simulink model "adc16_single_chan"  (R2013a)
settings: Solver=ode45  StartTime=0.0  StopTime=4096  RelTol=1e-3
undefined symbols (not defined in the file): pfb_coeff_gen_calc
libraries: xbsIndex_r4 x2131, casper_library_misc x50, simulink x31, casper_library_delays x18, casper_library_pfbs x4, xps_library x1
(part 1 of 27)
settings Model: Creator=root  LastModifiedBy=root

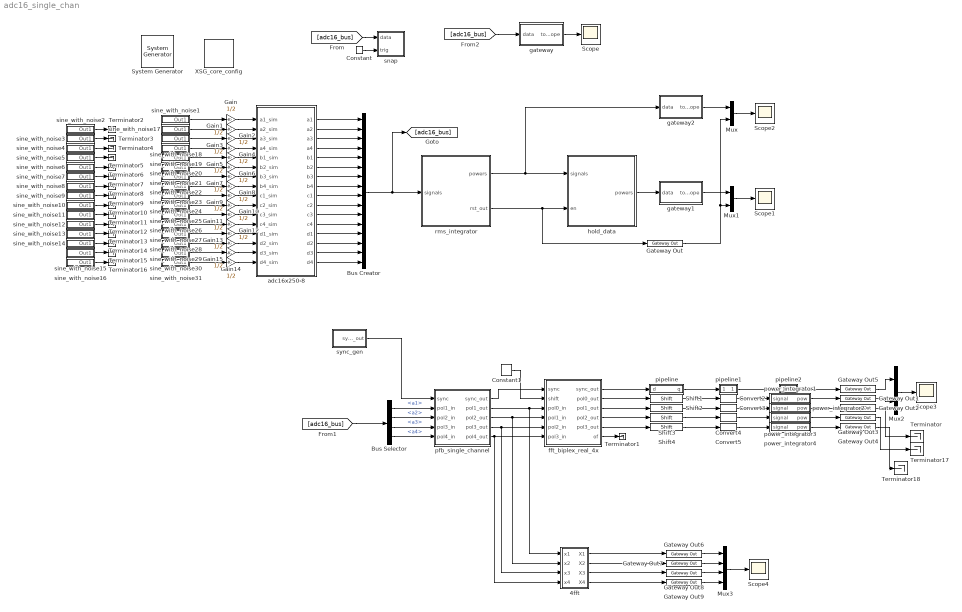
== system adc16_single_chan ==
  " System Generator" : xbsIndex_r4/ System Generator  Tag=genX  xilinxfamily=Kintex7  part=xc7k325t  speed=-3  package=fbg676  synthesis_tool=XST  clock_wrapper=Clock Enables  directory=./netlist  proj_type=Project Navigator  Synth_file=XST Defaults  Impl_file=ISE Defaults  testbench=off  simulink_period=1  sysclk_period=10  dcm_input_clock_period=10  incr_netlist=off  trim_vbits=Everywhere in SubSystem  dbl_ovrd=According to Block Masks  core_generation=According to Block Masks  run_coregen=off  deprecated_control=off  eval_field=0  block_type=sysgen
  4fft : Subsystem
  Bus Creator : BusCreator  Inputs=16
  Bus Selector : BusSelector  OutputSignals=a1,a2,a3,a4
  Constant : xbsIndex_r4/Constant  const=1  gui_display_data_type=Boolean  arith_type=Boolean  n_bits=16  bin_pt=14  preci_type=Single  exp_width=8  frac_width=24  explicit_period=off  period=1  equ=P=C  opselect=C  inp2=PCIN>>17  opr=+  inp1=P  carry=CIN  dbl_ovrd=off  block_type=constant
  Constant1 : xbsIndex_r4/Constant  const=3  gui_display_data_type=Fixed-point  arith_type=Unsigned  n_bits=2  bin_pt=0  preci_type=Single  exp_width=8  frac_width=24  explicit_period=on  period=1  equ=P=C  opselect=C  inp2=PCIN>>17  opr=+  inp1=P  carry=CIN  dbl_ovrd=off  block_type=constant
  Convert{2..5} (4 alike) : xbsIndex_r4/Convert  gui_display_data_type=Fixed-point  arith_type=Unsigned  n_bits=8  bin_pt=0  float_type=Single  exp_bits=8  fraction_bits=24  quantization=Truncate  overflow=Wrap  en=off  latency=2  dbl_ovrd=off  pipeline=off  block_type=convert
      settings: block_version=11.4
  Gain{,1..15} (16 alike) : Gain  Gain=1/2
  Gateway Out{,1..9} (10 alike) : xbsIndex_r4/Gateway Out  inherit_from_input=off  hdl_port=on  timing_constraint=None  locs_specified=off  LOCs={}  UseAsDAC=off  DACChannel='1'  block_type=gatewayout
  Mux : Mux  Inputs=2
  Mux1 : Mux  Inputs=2
  Mux2 : Mux  Inputs=2
  Mux3 : Mux
  Scope{,1..4} (5 alike) : Scope
      Scope2 settings: SaveName=ScopeData2
      Scope3 settings: SaveName=ScopeData3
      Scope4 settings: SaveName=ScopeData4
  Shift{1..4} (4 alike) : xbsIndex_r4/Shift  shift_dir=Right  shift_bits=27  en=off  latency=1  precision=Full  arith_type="Signed  (2's comp)"  n_bits=16  bin_pt=14  quantization=Truncate  overflow=Wrap  dbl_ovrd=off  block_type=shift
  Terminator{,1..18} (19 alike) : Terminator
  XSG_core_config : xps_library/XSG_core_config  Tag=xps:xsg  hw_sys=ROACH2:sx475t  clk_src=adc0_clk  ROACH_clk_src=sys_clk  ROACH2_clk_src=adc0_clk  MKDIG_clk_src=sys_clk  clk_rate=240  sample_period=1  synthesis_tool=XST
  adc16x250-8 : Subsystem  Tag=xps:adc16  AncestorBlock=xps_library/ADCs/adc16x250-8  mask(ADC16){board_count=1, roach2_rev=2, zdok_rev=2}
      mask prompts: board_count "Number of ADC16 Boards"; roach2_rev "ROACH2 Revision"; zdok_rev "ZDOK Pinout Revision"
      mask help: 16-input ADC. When using one ADC16 board, it must be in ZDOK0.
      mask init:
      | % Only board_count is needed by init function
      | adc16_init(gcb, ...
      |     'board_count', board_count);
      settings: AttributesFormatString=r2 rev%<roach2_rev>\nzdok rev%<zdok_rev>
      mask Help:
      | This is the CASPER "yellow block" for the CASPER ADC16 board.  Each ADC
      | board has four ADC chips.  Each ADC chip accepts four inputs.  The four
      | 8-bit outputs from each ADC chip are concatenated into a 32-bit signal.
      mask TypeOptions board_count: 1 | 2
      mask TypeOptions roach2_rev: 1 | 2
      mask TypeOptions zdok_rev: 1 | 2
  fft_biplex_real_4x : Subsystem  Tag=casper:fft_biplex_real_4x  AncestorBlock=casper_library_ffts/fft_biplex_real_4x  mask(fft_biplex_real_4x){n_inputs=1, FFTSize=2, input_bit_width=18, bin_pt_in=17, coeff_bit_width=18, async=off, add_latency=1, mult_latency=2, bram_latency=2, conv_latency=1, quantization=Round  (unbiased: +/- Inf), overflow=Saturate, delays_bit_limit=8, coeffs_bit_limit=8, coeff_sharing=on, coeff_decimation=on, max_fanout=4, mult_spec=2, bitgrowth=off, max_bits=19, hardcode_shifts=off, shift_schedule=[1                                      1], dsp48_adders=off}
      mask prompts: n_inputs "Number simultaneous inputs (4*?)"; FFTSize "Size of FFT: (2^? pts)"; input_bit_width "Input bit width"; bin_pt_in "Input binary point"; coeff_bit_width "Coefficient Bit Width"; async "Asynchronous operation"; add_latency "Add Latency"; mult_latency "Mult Latency"; bram_latency "BRAM Latency"; conv_latency "Convert latency"; quantization "Quantization Behavior"; overflow "Overflow Behavior"; delays_bit_limit "Number bits above which to implement stage's delays in BRAM (2^? bits)"; coeffs_bit_limit "Number bits above which to store stage's coefficients in BRAM (2^? bits)"; coeff_sharing "BRAM sharing in coeff storage"; coeff_decimation "Store a fraction of coeff factors where useful"; max_fanout "Maximum fanout"; mult_spec "Multiplier impl. (0=core, 1=embedded, 2=behavioural) (left=1st stage, or just one value)"; bitgrowth "Bitgrowth instead of shifting"; max_bits "Max bits to grow to"; hardcode_shifts "Hardcode shift schedule"; shift_schedule "Shift schedule"; dsp48_adders "DSP48 adders in butterfly"
      mask help: A real-sampled biplex FFT, with output demuxed by 4.
      mask init:
      | fft_biplex_real_4x_init(gcb, ...
      |     'n_inputs', n_inputs, ...
      |     'FFTSize', FFTSize, ...
      |     'input_bit_width', input_bit_width, ...
      |     'bin_pt_in', bin_pt_in, ...
      |     'coeff_bit_width', coeff_bit_width, ...
      |     'async', async, ...
      |     'add_latency', add_latency, ...
      |     'mult_latency', mult_latency, ...
      |     'bram_latency', bram_latency, ...
      |     'conv_latency', conv_latency, ...
      |     'quantization', quantization, ...
      |     'overflow', overflow, ...
      |     'delays_bit_limit', delays_bit_limit, ... 
      |     'coeffs_bit_limit', coeffs_bit_limit, ...
      |     'coeff_sharing', coeff_sharing, ...
      |     'coeff_decimation', coeff_decimation, ...
      |     'max_fanout', max_fanout, ...   
      |     'mult_spec', mult_spec, ...
      |     'bitgrowth', bitgrowth, ...
      |     'max_bits', max_bits, ...
      |     'hardcode_shifts', hardcode_shifts, ...
      |     'shift_schedule', shift_schedule, ...
      |     'dsp48_adders', dsp48_adders);
      settings: AttributesFormatString=|
      | 2 stages
      | [18,18]
      | Round  (unbiased: +/- Inf)
      | Saturate
      mask Help: eval('xlWeb(''http://casper.berkeley.edu/wiki/Fft_biplex_real_4x'')')
      mask TypeOptions quantization: Truncate | Round  (unbiased: +/- Inf) | Round  (unbiased: Even Values)
      mask TypeOptions overflow: Wrap | Saturate | Error
      mask Callback hardcode_shifts:
      | hardcode_shifts = get_param(gcb, 'hardcode_shifts');
      | set_param_state(gcb, 'shift_schedule', hardcode_shifts);
      mask Callback dsp48_adders: fft_callback_dsp48_adders(gcb);
  gateway : Subsystem
  gateway1 : Subsystem
  gateway2 : Subsystem
  hold_data : Subsystem
  pfb_single_channel : Subsystem
  pipeline : Subsystem  AncestorBlock=casper_library_delays/pipeline  mask(pipeline){latency=1}
      mask help:
      | An explicitly laid-out delay line to avoid mapping to SRL16s
      | for use in pipelining to help achieve timing closure.
      mask init:
      | pipeline_init(gcb,'latency',latency);
      settings: AttributesFormatString=Latency = %<latency>
      mask Display:
      | port_label('input', 1, 'd');
      | port_label('output', 1, 'q');
      | disp(['Z^-', num2str(latency)]);
  pipeline1 : Subsystem  AncestorBlock=casper_library_delays/pipeline  mask(pipeline){latency=2}
      mask help:
      | An explicitly laid-out delay line to avoid mapping to SRL16s
      | for use in pipelining to help achieve timing closure.
      mask init:
      | pipeline_init(gcb,'latency',latency);
      settings: AttributesFormatString=Latency = %<latency>
      mask Display:
      | port_label('input', 1, 'd');
      | port_label('output', 1, 'q');
      | disp(['Z^-', num2str(latency)]);
  pipeline2 : Subsystem  AncestorBlock=casper_library_delays/pipeline  mask(pipeline){latency=5}
      mask help:
      | An explicitly laid-out delay line to avoid mapping to SRL16s
      | for use in pipelining to help achieve timing closure.
      mask init:
      | pipeline_init(gcb,'latency',latency);
      settings: AttributesFormatString=Latency = %<latency>
      mask Display:
      | port_label('input', 1, 'd');
      | port_label('output', 1, 'q');
      | disp(['Z^-', num2str(latency)]);
  power_integrator1 : Subsystem
  power_integrator2 : Subsystem
  power_integrator3 : Subsystem
  power_integrator4 : Subsystem
  rms_integrator : Subsystem
  sine_with_noise1 : Subsystem
  sine_with_noise10 : Subsystem
  sine_with_noise11 : Subsystem
  sine_with_noise12 : Subsystem
  sine_with_noise13 : Subsystem
  sine_with_noise14 : Subsystem
  sine_with_noise15 : Subsystem
  sine_with_noise16 : Subsystem
  sine_with_noise17 : Subsystem
  sine_with_noise18 : Subsystem
  sine_with_noise19 : Subsystem
  sine_with_noise2 : Subsystem
  sine_with_noise20 : Subsystem
  sine_with_noise21 : Subsystem
  sine_with_noise22 : Subsystem
  sine_with_noise23 : Subsystem
  sine_with_noise24 : Subsystem
  sine_with_noise25 : Subsystem
  sine_with_noise26 : Subsystem
  sine_with_noise27 : Subsystem
  sine_with_noise28 : Subsystem
  sine_with_noise29 : Subsystem
  sine_with_noise3 : Subsystem
  sine_with_noise30 : Subsystem
  sine_with_noise31 : Subsystem
  sine_with_noise4 : Subsystem
  sine_with_noise5 : Subsystem
  sine_with_noise6 : Subsystem
  sine_with_noise7 : Subsystem
  sine_with_noise8 : Subsystem
  sine_with_noise9 : Subsystem
  snap : Subsystem
  sync_gen : Subsystem  AncestorBlock=casper_library_misc/sync_gen  mask(sync_gen){sim_acc_len=4, fft_size=4, fft_simult_inputs=1, pfb_fir_taps=1, reorder_vec=[2 2 2], scale=32}
      mask prompts: sim_acc_len "Simulation Accumulation Length"; fft_size "FFT Size"; fft_simult_inputs "Simultaneous Inputs (FFT)"; pfb_fir_taps "Taps in pfb_fir (use 1 if no pfb_fir)"; reorder_vec "Reorder Orders (e.g. [2 2 2])"
      mask help:
      | This block computes the sync period based on system parameters as
      | described in Casper memo.  Detailed descritions of the block's
      | variables can be found in the 'Block Documentation' section of
      | the CASPER wiki.
      mask init:
      | sync_gen_init(gcb, ...
      |     'sim_acc_len', sim_acc_len, ...
      |     'fft_size', fft_size, ...
      |     'fft_simult_inputs', fft_simult_inputs,...
      |     'pfb_fir_taps', pfb_fir_taps, ...
      |     'reorder_vec', reorder_vec, ...
      |     'scale', scale);
      settings: AttributesFormatString=sim_sync_period=1024
      mask Help:
      | SyncPeriod=LCM(reorder_vec)*(acc_num)*(pfb_fir_len)*(fft_size/fft_simult_inputs)
      | 
      | See CASPER sync pulse memo for more details.
  wires:
  adc16x250-8/15(d3) -> Bus Creator/15
  adc16x250-8/16(d4) -> Bus Creator/16
  adc16x250-8/12(c4) -> Bus Creator/12
  adc16x250-8/3(a3) -> Bus Creator/3
  adc16x250-8/13(d1) -> Bus Creator/13
  adc16x250-8/5(b1) -> Bus Creator/5
  adc16x250-8/10(c2) -> Bus Creator/10
  adc16x250-8/8(b4) -> Bus Creator/8
  adc16x250-8/2(a2) -> Bus Creator/2
  adc16x250-8/11(c3) -> Bus Creator/11
  adc16x250-8/7(b3) -> Bus Creator/7
  adc16x250-8/14(d2) -> Bus Creator/14
  adc16x250-8/9(c1) -> Bus Creator/9
  adc16x250-8/4(a4) -> Bus Creator/4
  adc16x250-8/6(b2) -> Bus Creator/6
  [adc16_bus] -> snap/1(data)
  Constant/1 -> snap/2(trig)
  gateway/1(to_scope) -> Scope/1
  sine_with_noise1/1(Out1) -> Gain/1
  Gain/1 -> adc16x250-8/1(a1_sim)
  Gain1/1 -> adc16x250-8/2(a2_sim)
  Gain2/1 -> adc16x250-8/3(a3_sim)
  Gain3/1 -> adc16x250-8/4(a4_sim)
  Gain4/1 -> adc16x250-8/5(b1_sim)
  Gain5/1 -> adc16x250-8/6(b2_sim)
  Gain6/1 -> adc16x250-8/7(b3_sim)
  Gain7/1 -> adc16x250-8/8(b4_sim)
  Gain10/1 -> adc16x250-8/11(c3_sim)
  Gain8/1 -> adc16x250-8/9(c1_sim)
  Gain12/1 -> adc16x250-8/13(d1_sim)
  Gain15/1 -> adc16x250-8/16(d4_sim)
  Gain11/1 -> adc16x250-8/12(c4_sim)
  Gain14/1 -> adc16x250-8/15(d3_sim)
  Gain9/1 -> adc16x250-8/10(c2_sim)
  Gain13/1 -> adc16x250-8/14(d2_sim)
  adc16x250-8/1(a1) -> Bus Creator/1
  Bus Creator/1 -> [adc16_bus], rms_integrator/1(signals)
  rms_integrator/1(powers) -> gateway2/1(data), hold_data/1(signals)
  hold_data/1(powers) -> gateway1/1(data)
  gateway2/1(to_scope) -> Mux/1
  Mux/1 -> Scope2/1
  rms_integrator/2(rst_out) -> Gateway Out/1, hold_data/2(en)
  gateway1/1(to_scope) -> Mux1/1
  Mux1/1 -> Scope1/1
  Gateway Out/1 -> Mux/2, Mux1/2
  [adc16_bus] -> Bus Selector/1
  [adc16_bus] -> gateway/1(data)
  Constant1/1 -> fft_biplex_real_4x/2(shift)
  fft_biplex_real_4x/1(sync_out) -> pipeline/1(d)
  fft_biplex_real_4x/6(of) -> Terminator1/1
  fft_biplex_real_4x/5(pol3_out) -> Shift4/1
  fft_biplex_real_4x/2(pol0_out) -> Shift1/1
  fft_biplex_real_4x/3(pol1_out) -> Shift2/1
  fft_biplex_real_4x/4(pol2_out) -> Shift3/1
  Mux2/1 -> Scope3/1
  sync_gen/1(sync_out) -> pfb_single_channel/1(sync)
  pfb_single_channel/1(sync_out) -> fft_biplex_real_4x/1(sync)
  pfb_single_channel/2(pol1_out) -> 4fft/1(x1), fft_biplex_real_4x/3(pol0_in)
  pfb_single_channel/4(pol3_out) -> 4fft/3(x3), fft_biplex_real_4x/5(pol2_in)
  pfb_single_channel/3(pol2_out) -> 4fft/2(x2), fft_biplex_real_4x/4(pol1_in)
  pfb_single_channel/5(pol4_out) -> 4fft/4(x4), fft_biplex_real_4x/6(pol3_in)
  Bus Selector/4 -> pfb_single_channel/5(pol4_in)  "<a4>"
  Bus Selector/2 -> pfb_single_channel/3(pol2_in)  "<a2>"
  Bus Selector/1 -> pfb_single_channel/2(pol1_in)  "<a1>"
  Bus Selector/3 -> pfb_single_channel/4(pol3_in)  "<a3>"
  Shift1/1 -> Convert2/1
  Shift2/1 -> Convert3/1
  Shift3/1 -> Convert4/1
  Shift4/1 -> Convert5/1
  Gateway Out1/1 -> Mux2/2
  Gateway Out5/1 -> Mux2/1
  pipeline/1(q) -> pipeline1/1(d)
  Convert2/1 -> power_integrator1/1(signal)
  Convert3/1 -> power_integrator2/1(signal)
  Convert4/1 -> power_integrator3/1(signal)
  Convert5/1 -> power_integrator4/1(signal)
  pipeline1/1(q) -> pipeline2/1(d)
  power_integrator1/1(pow) -> Gateway Out1/1
  power_integrator2/1(pow) -> Gateway Out2/1
  power_integrator3/1(pow) -> Gateway Out3/1
  power_integrator4/1(pow) -> Gateway Out4/1
  sine_with_noise17/1(Out1) -> Gain1/1
  sine_with_noise18/1(Out1) -> Gain2/1
  sine_with_noise19/1(Out1) -> Gain3/1
  sine_with_noise20/1(Out1) -> Gain4/1
  sine_with_noise21/1(Out1) -> Gain5/1
  sine_with_noise22/1(Out1) -> Gain6/1
  sine_with_noise23/1(Out1) -> Gain7/1
  sine_with_noise24/1(Out1) -> Gain8/1
  sine_with_noise25/1(Out1) -> Gain9/1
  sine_with_noise26/1(Out1) -> Gain10/1
  sine_with_noise27/1(Out1) -> Gain11/1
  sine_with_noise28/1(Out1) -> Gain12/1
  sine_with_noise29/1(Out1) -> Gain13/1
  sine_with_noise30/1(Out1) -> Gain14/1
  sine_with_noise31/1(Out1) -> Gain15/1
  sine_with_noise2/1(Out1) -> Terminator2/1
  sine_with_noise3/1(Out1) -> Terminator3/1
  sine_with_noise4/1(Out1) -> Terminator4/1
  sine_with_noise5/1(Out1) -> Terminator5/1
  sine_with_noise6/1(Out1) -> Terminator6/1
  sine_with_noise7/1(Out1) -> Terminator7/1
  sine_with_noise8/1(Out1) -> Terminator8/1
  sine_with_noise9/1(Out1) -> Terminator9/1
  sine_with_noise10/1(Out1) -> Terminator10/1
  sine_with_noise11/1(Out1) -> Terminator11/1
  sine_with_noise12/1(Out1) -> Terminator12/1
  sine_with_noise13/1(Out1) -> Terminator13/1
  sine_with_noise14/1(Out1) -> Terminator14/1
  sine_with_noise15/1(Out1) -> Terminator15/1
  sine_with_noise16/1(Out1) -> Terminator16/1
  pipeline2/1(q) -> Gateway Out5/1
  Gateway Out2/1 -> Terminator/1
  Gateway Out3/1 -> Terminator17/1
  Gateway Out4/1 -> Terminator18/1
  4fft/3(X3) -> Gateway Out8/1
  4fft/4(X4) -> Gateway Out9/1
  4fft/2(X2) -> Gateway Out7/1
  4fft/1(X1) -> Gateway Out6/1
  Gateway Out9/1 -> Mux3/4
  Gateway Out7/1 -> Mux3/2
  Gateway Out6/1 -> Mux3/1
  Gateway Out8/1 -> Mux3/3
  Mux3/1 -> Scope4/1

== system adc16_single_chan/4fft ==
  x1 : Inport
  x2 : Inport  Port=2
  x3 : Inport  Port=3
  x4 : Inport  Port=4
  AddSub{,1,4..7} (6 alike) : xbsIndex_r4/AddSub  mode=Addition  use_carryin=off  use_carryout=off  en=off  latency=0  precision=Full  arith_type=Unsigned  n_bits=16  bin_pt=14  quantization=Truncate  overflow=Wrap  dbl_ovrd=off  use_behavioral_HDL=off  hw_selection=Fabric  pipelined=off  block_type=addsub
  AddSub2 : xbsIndex_r4/AddSub  mode=Subtraction  use_carryin=off  use_carryout=off  en=off  latency=0  precision=Full  arith_type=Unsigned  n_bits=16  bin_pt=14  quantization=Truncate  overflow=Wrap  dbl_ovrd=off  use_behavioral_HDL=off  hw_selection=Fabric  pipelined=off  block_type=addsub
  AddSub3 : xbsIndex_r4/AddSub  mode=Subtraction  use_carryin=off  use_carryout=off  en=off  latency=0  precision=Full  arith_type=Unsigned  n_bits=16  bin_pt=14  quantization=Truncate  overflow=Wrap  dbl_ovrd=off  use_behavioral_HDL=off  hw_selection=Fabric  pipelined=off  block_type=addsub
  Negate2 : xbsIndex_r4/Negate  precision=User Defined  arith_type="Signed  (2's comp)"  n_bits=19  bin_pt=17  quantization=Truncate  overflow=Wrap  en=off  latency=0  dbl_ovrd=off  block_type=negate
  mult_j : Subsystem
  mult_jjj : Subsystem
  X1 : Outport
  X2 : Outport  Port=2
  X3 : Outport  Port=3
  X4 : Outport  Port=4
  wires:
  x1/1 -> AddSub2/1, AddSub/1
  x2/1 -> AddSub3/1, AddSub1/1
  AddSub1/1 -> Negate2/1, AddSub4/2
  Negate2/1 -> AddSub5/2
  AddSub/1 -> AddSub5/1, AddSub4/1
  AddSub2/1 -> AddSub7/1, AddSub6/1
  AddSub4/1 -> X1/1
  AddSub5/1 -> X3/1
  AddSub6/1 -> X2/1
  AddSub7/1 -> X4/1
  AddSub3/1 -> mult_jjj/1(a+jb), mult_j/1(a+jb)
  mult_j/1(ja-b) -> AddSub7/2
  mult_jjj/1(b-ja) -> AddSub6/2
  x4/1 -> AddSub3/2, AddSub1/2
  x3/1 -> AddSub2/2, AddSub/2

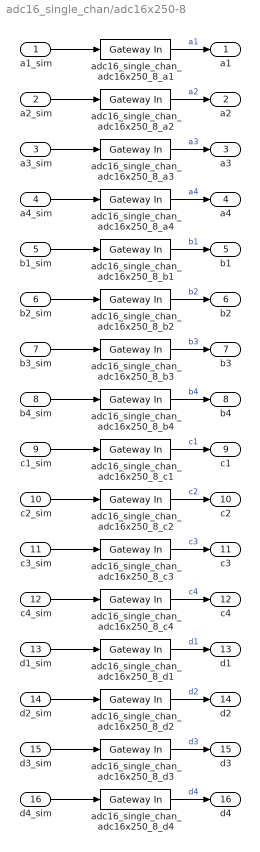
== system adc16_single_chan/adc16x250-8 ==
  a1_sim : Inport
  a2_sim : Inport  Port=2
  a3_sim : Inport  Port=3
  a4_sim : Inport  Port=4
  b1_sim : Inport  Port=5
  b2_sim : Inport  Port=6
  b3_sim : Inport  Port=7
  b4_sim : Inport  Port=8
  c1_sim : Inport  Port=9
  c2_sim : Inport  Port=10
  c3_sim : Inport  Port=11
  c4_sim : Inport  Port=12
  d1_sim : Inport  Port=13
  d2_sim : Inport  Port=14
  d3_sim : Inport  Port=15
  d4_sim : Inport  Port=16
  adc16_single_chan_adc16x250_8_a{1..4} (4 alike) : xbsIndex_r4/Gateway In  gui_display_data_type=Fixed-point  arith_type="Signed  (2's comp)"  n_bits=8  bin_pt=7  preci_type=Single  exp_width=8  frac_width=24  quantization="Round  (unbiased: +/- Inf)"  overflow=Saturate  period=1  dbl_ovrd=off  timing_constraint=None  locs_specified=off  LOCs={}  UseAsADC=off  ADCChannel='1'  inherit_from_input=off  hdl_port=on  block_type=gatewayin
  adc16_single_chan_adc16x250_8_b{1..4} (4 alike) : xbsIndex_r4/Gateway In  gui_display_data_type=Fixed-point  arith_type="Signed  (2's comp)"  n_bits=8  bin_pt=7  preci_type=Single  exp_width=8  frac_width=24  quantization="Round  (unbiased: +/- Inf)"  overflow=Saturate  period=1  dbl_ovrd=off  timing_constraint=None  locs_specified=off  LOCs={}  UseAsADC=off  ADCChannel='1'  inherit_from_input=off  hdl_port=on  block_type=gatewayin
  adc16_single_chan_adc16x250_8_c{1..4} (4 alike) : xbsIndex_r4/Gateway In  gui_display_data_type=Fixed-point  arith_type="Signed  (2's comp)"  n_bits=8  bin_pt=7  preci_type=Single  exp_width=8  frac_width=24  quantization="Round  (unbiased: +/- Inf)"  overflow=Saturate  period=1  dbl_ovrd=off  timing_constraint=None  locs_specified=off  LOCs={}  UseAsADC=off  ADCChannel='1'  inherit_from_input=off  hdl_port=on  block_type=gatewayin
  adc16_single_chan_adc16x250_8_d{1..4} (4 alike) : xbsIndex_r4/Gateway In  gui_display_data_type=Fixed-point  arith_type="Signed  (2's comp)"  n_bits=8  bin_pt=7  preci_type=Single  exp_width=8  frac_width=24  quantization="Round  (unbiased: +/- Inf)"  overflow=Saturate  period=1  dbl_ovrd=off  timing_constraint=None  locs_specified=off  LOCs={}  UseAsADC=off  ADCChannel='1'  inherit_from_input=off  hdl_port=on  block_type=gatewayin
  a1 : Outport
  a2 : Outport  Port=2
  a3 : Outport  Port=3
  a4 : Outport  Port=4
  b1 : Outport  Port=5
  b2 : Outport  Port=6
  b3 : Outport  Port=7
  b4 : Outport  Port=8
  c1 : Outport  Port=9
  c2 : Outport  Port=10
  c3 : Outport  Port=11
  c4 : Outport  Port=12
  d1 : Outport  Port=13
  d2 : Outport  Port=14
  d3 : Outport  Port=15
  d4 : Outport  Port=16
  wires:
  a1_sim/1 -> adc16_single_chan_adc16x250_8_a1/1
  adc16_single_chan_adc16x250_8_a1/1 -> a1/1  "a1"
  a2_sim/1 -> adc16_single_chan_adc16x250_8_a2/1
  adc16_single_chan_adc16x250_8_a2/1 -> a2/1  "a2"
  a3_sim/1 -> adc16_single_chan_adc16x250_8_a3/1
  adc16_single_chan_adc16x250_8_a3/1 -> a3/1  "a3"
  a4_sim/1 -> adc16_single_chan_adc16x250_8_a4/1
  adc16_single_chan_adc16x250_8_a4/1 -> a4/1  "a4"
  b1_sim/1 -> adc16_single_chan_adc16x250_8_b1/1
  adc16_single_chan_adc16x250_8_b1/1 -> b1/1  "b1"
  b2_sim/1 -> adc16_single_chan_adc16x250_8_b2/1
  adc16_single_chan_adc16x250_8_b2/1 -> b2/1  "b2"
  b3_sim/1 -> adc16_single_chan_adc16x250_8_b3/1
  adc16_single_chan_adc16x250_8_b3/1 -> b3/1  "b3"
  b4_sim/1 -> adc16_single_chan_adc16x250_8_b4/1
  adc16_single_chan_adc16x250_8_b4/1 -> b4/1  "b4"
  c1_sim/1 -> adc16_single_chan_adc16x250_8_c1/1
  adc16_single_chan_adc16x250_8_c1/1 -> c1/1  "c1"
  c2_sim/1 -> adc16_single_chan_adc16x250_8_c2/1
  adc16_single_chan_adc16x250_8_c2/1 -> c2/1  "c2"
  c3_sim/1 -> adc16_single_chan_adc16x250_8_c3/1
  adc16_single_chan_adc16x250_8_c3/1 -> c3/1  "c3"
  c4_sim/1 -> adc16_single_chan_adc16x250_8_c4/1
  adc16_single_chan_adc16x250_8_c4/1 -> c4/1  "c4"
  d1_sim/1 -> adc16_single_chan_adc16x250_8_d1/1
  adc16_single_chan_adc16x250_8_d1/1 -> d1/1  "d1"
  d2_sim/1 -> adc16_single_chan_adc16x250_8_d2/1
  adc16_single_chan_adc16x250_8_d2/1 -> d2/1  "d2"
  d3_sim/1 -> adc16_single_chan_adc16x250_8_d3/1
  adc16_single_chan_adc16x250_8_d3/1 -> d3/1  "d3"
  d4_sim/1 -> adc16_single_chan_adc16x250_8_d4/1
  adc16_single_chan_adc16x250_8_d4/1 -> d4/1  "d4"

== system adc16_single_chan/fft_biplex_real_4x ==
  sync : Inport
  shift : Inport  Port=2
  pol0_in : Inport  Port=3
  pol1_in : Inport  Port=4
  pol2_in : Inport  Port=5
  pol3_in : Inport  Port=6
  bi_real_unscr_4x : Subsystem  AncestorBlock=casper_library_ffts_internal/bi_real_unscr_4x  mask(bi_real_unscr_4x){n_inputs=1, FFTSize=2, n_bits=18, bin_pt=17, add_latency=add_latency, conv_latency=conv_latency, bram_latency=bram_latency, bram_map=off, bram_delays=off, dsp48_adders=off, async=off}
      mask prompts: n_inputs "Number simultaneous inputs (2*?)"; FFTSize "Size of FFT (2^?):"; n_bits "Sample Bit Width"; bin_pt "Sample binary point"; add_latency "Add Latency"; conv_latency "Convert Latency"; bram_latency "BRAM Latency"; bram_map "Use BlockRAM for Map"; bram_delays "Use BlockRAM for Delays"; dsp48_adders "Use DSP48s for adders"; async "Asynchonrous operation"
      mask help: FFT internal block.
      mask init:
      | bi_real_unscr_4x_init(gcb, ...
      |     'n_inputs', n_inputs, ...
      |     'FFTSize', FFTSize, ...
      |     'n_bits', n_bits, ...
      |     'bin_pt', bin_pt, ...
      |     'add_latency', add_latency, ...
      |     'conv_latency', conv_latency, ...
      |     'bram_latency', bram_latency, ...
      |     'bram_map', bram_map, ...
      |     'bram_delays', bram_delays, ...
      |     'dsp48_adders', dsp48_adders, ...
      |     'async', async);
  biplex_core : Subsystem  AncestorBlock=casper_library_ffts/biplex_core  mask(biplex_core){n_inputs=1, FFTSize=2, input_bit_width=18, bin_pt_in=17, coeff_bit_width=18, add_latency=1, mult_latency=2, bram_latency=2, conv_latency=1, quantization=Round  (unbiased: +/- Inf), overflow=Saturate, delays_bit_limit=8, coeffs_bit_limit=8, coeff_sharing=on, coeff_decimation=on, max_fanout=4, mult_spec=[2 2], bitgrowth=off, max_bits=19, hardcode_shifts=off, shift_schedule=[1 1], dsp48_adders=off, async=off}
      mask prompts: n_inputs "Number inputs (2*?)"; FFTSize "Size of FFT: (2^? pts)"; input_bit_width "Input Bit Width"; bin_pt_in "Input binary point"; coeff_bit_width "Coefficient Bit Width"; add_latency "Add Latency"; mult_latency "Mult Latency"; bram_latency "BRAM Latency"; conv_latency "Convert latency"; quantization "Quantization Behavior"; overflow "Overflow Behavior"; delays_bit_limit "Number bits above which to implent stage's delays in BRAM (2^? bits)"; coeffs_bit_limit "Number bits above which to store stage's coefficients in BRAM (2^? bits)"; coeff_sharing "BRAM sharing in coeff storage"; coeff_decimation "Store a fraction of coeff factors where useful"; max_fanout "Maximum fanout"; mult_spec "Multiplier impl. (0=core, 1=embedded, 2=behavioural) (left=1st stage, or just one value)"; bitgrowth "Bit growth instead of shift"; max_bits "Maximum number of bits"; hardcode_shifts "Hardcode shift schedule"; shift_schedule "Shift schedule"; dsp48_adders "Use DSP48s for adders"; async "Asynchronous operation"
      mask help: FFT internal block.
      mask init:
      | biplex_core_init(gcb, ...
      |     'n_inputs', n_inputs, ...
      |     'FFTSize', FFTSize,...
      |     'input_bit_width', input_bit_width,...
      |     'bin_pt_in', bin_pt_in,...
      |     'coeff_bit_width', coeff_bit_width,...
      |     'async', async, ...
      |     'add_latency', add_latency,...
      |     'mult_latency', mult_latency,...
      |     'bram_latency', bram_latency,...
      |     'conv_latency', conv_latency, ...
      |     'quantization', quantization,...
      |     'overflow', overflow,...
      |     'delays_bit_limit', delays_bit_limit, ...
      |     'coeffs_bit_limit', coeffs_bit_limit, ...
      |     'coeff_sharing', coeff_sharing, ...
      |     'coeff_decimation', coeff_decimation, ...
      |     'max_fanout', max_fanout, ...
      |     'mult_spec', mult_spec, ...
      |     'bitgrowth', bitgrowth, ...
      |     'max_bits', max_bits, ...
      |     'hardcode_shifts', hardcode_shifts, ...
      |     'shift_schedule', shift_schedule, ...
      |     'dsp48_adders', dsp48_adders);
      settings: AttributesFormatString=2 stages
      mask TypeOptions quantization: Truncate | Round  (unbiased: +/- Inf) | Round  (unbiased: Even Values)
      mask TypeOptions overflow: Wrap | Saturate | Error
      mask Callback hardcode_shifts:
      | hardcode_shifts = get_param(gcb, 'hardcode_shifts');
      | set_param_state(gcb, 'shift_schedule', hardcode_shifts);
      mask Callback dsp48_adders: fft_callback_dsp48_adders(gcb);
  even_bussify : Subsystem  AncestorBlock=casper_library_flow_control/bus_create  mask(bus_create){inputNum=1}
      mask prompts: inputNum "Number of inputs:"
      mask init:
      | bus_create_init(gcb,...
      |     'inputNum', inputNum);
  odd_bussify : Subsystem  AncestorBlock=casper_library_flow_control/bus_create  mask(bus_create){inputNum=1}
      mask prompts: inputNum "Number of inputs:"
      mask init:
      | bus_create_init(gcb,...
      |     'inputNum', inputNum);
  pol0_debus : Subsystem  AncestorBlock=casper_library_flow_control/bus_expand  mask(bus_expand){mode=divisions of equal size, outputNum=1, outputWidth=36, outputBinaryPt=0, outputArithmeticType=0, show_format=off, outputToWorkspace=off, variablePrefix=out, outputToModelAsWell=on}
      mask prompts: outputNum "Number of outputs:"; outputWidth "Output width:"; outputBinaryPt "Output binary point position:"; outputArithmeticType "Output arithmetic type (ufix=0, fix=1, bool=2):"; show_format "Print format string?"; outputToWorkspace "Output to workspace?"; variablePrefix "Variable name prefix:"; outputToModelAsWell "Output to model as well?"
      mask help:
      | Expands a 'bus' made using a bus_create or Xilinx
      | concat block.
      | The input will be divided into the specified number
      | of outputs with the specified arithmetic types.
      | Divisions are made from most significant bit.
      mask init:
      | bus_expand_init(gcb,...
      |     'mode', mode, ...
      |     'outputNum', outputNum, ...
      |     'outputWidth', outputWidth, ...
      |     'outputBinaryPt', outputBinaryPt, ...
      |     'outputArithmeticType', outputArithmeticType, ...
      |     'show_format', show_format, ...
      |     'outputToWorkspace', outputToWorkspace, ...
      |     'variablePrefix', variablePrefix, ...
      |     'outputToModelAsWell', outputToModelAsWell);
      settings: AttributesFormatString=1 outputs
      mask TypeOptions mode: divisions of equal size | divisions of arbitrary size
      mask Callback mode: bus_expand_callback();
      mask Callback outputWidth: bus_expand_callback();
      mask Callback outputToWorkspace: bus_expand_callback();
  pol1_debus : Subsystem  AncestorBlock=casper_library_flow_control/bus_expand  mask(bus_expand){mode=divisions of equal size, outputNum=1, outputWidth=36, outputBinaryPt=0, outputArithmeticType=0, show_format=off, outputToWorkspace=off, variablePrefix=out, outputToModelAsWell=on}
      mask prompts: outputNum "Number of outputs:"; outputWidth "Output width:"; outputBinaryPt "Output binary point position:"; outputArithmeticType "Output arithmetic type (ufix=0, fix=1, bool=2):"; show_format "Print format string?"; outputToWorkspace "Output to workspace?"; variablePrefix "Variable name prefix:"; outputToModelAsWell "Output to model as well?"
      mask help:
      | Expands a 'bus' made using a bus_create or Xilinx
      | concat block.
      | The input will be divided into the specified number
      | of outputs with the specified arithmetic types.
      | Divisions are made from most significant bit.
      mask init: same as adc16_single_chan/fft_biplex_real_4x/pol0_debus
      settings: AttributesFormatString=1 outputs
      mask TypeOptions mode: divisions of equal size | divisions of arbitrary size
      mask Callback mode: bus_expand_callback();
      mask Callback outputWidth: bus_expand_callback();
      mask Callback outputToWorkspace: bus_expand_callback();
  pol2_debus : Subsystem  AncestorBlock=casper_library_flow_control/bus_expand  mask(bus_expand){mode=divisions of equal size, outputNum=1, outputWidth=36, outputBinaryPt=0, outputArithmeticType=0, show_format=off, outputToWorkspace=off, variablePrefix=out, outputToModelAsWell=on}
      mask prompts: outputNum "Number of outputs:"; outputWidth "Output width:"; outputBinaryPt "Output binary point position:"; outputArithmeticType "Output arithmetic type (ufix=0, fix=1, bool=2):"; show_format "Print format string?"; outputToWorkspace "Output to workspace?"; variablePrefix "Variable name prefix:"; outputToModelAsWell "Output to model as well?"
      mask help:
      | Expands a 'bus' made using a bus_create or Xilinx
      | concat block.
      | The input will be divided into the specified number
      | of outputs with the specified arithmetic types.
      | Divisions are made from most significant bit.
      mask init: same as adc16_single_chan/fft_biplex_real_4x/pol0_debus
      settings: AttributesFormatString=1 outputs
      mask TypeOptions mode: divisions of equal size | divisions of arbitrary size
      mask Callback mode: bus_expand_callback();
      mask Callback outputWidth: bus_expand_callback();
      mask Callback outputToWorkspace: bus_expand_callback();
  pol3_debus : Subsystem  AncestorBlock=casper_library_flow_control/bus_expand  mask(bus_expand){mode=divisions of equal size, outputNum=1, outputWidth=36, outputBinaryPt=0, outputArithmeticType=0, show_format=off, outputToWorkspace=off, variablePrefix=out, outputToModelAsWell=on}
      mask prompts: outputNum "Number of outputs:"; outputWidth "Output width:"; outputBinaryPt "Output binary point position:"; outputArithmeticType "Output arithmetic type (ufix=0, fix=1, bool=2):"; show_format "Print format string?"; outputToWorkspace "Output to workspace?"; variablePrefix "Variable name prefix:"; outputToModelAsWell "Output to model as well?"
      mask help:
      | Expands a 'bus' made using a bus_create or Xilinx
      | concat block.
      | The input will be divided into the specified number
      | of outputs with the specified arithmetic types.
      | Divisions are made from most significant bit.
      mask init: same as adc16_single_chan/fft_biplex_real_4x/pol0_debus
      settings: AttributesFormatString=1 outputs
      mask TypeOptions mode: divisions of equal size | divisions of arbitrary size
      mask Callback mode: bus_expand_callback();
      mask Callback outputWidth: bus_expand_callback();
      mask Callback outputToWorkspace: bus_expand_callback();
  ri_to_c0 : Subsystem  AncestorBlock=casper_library_misc/ri_to_c  mask(ri_to_c){}
      mask help:
      | Concatenates real and imaginary inputs into a complex output.
      | Useful for simplifying interconnects.
      | See also: Complex to Real-Imag (c_to_ri)
      mask Help: eval('xlWeb(''http://casper.berkeley.edu/wiki/Ri_to_c'')')
  ri_to_c1 : Subsystem  AncestorBlock=casper_library_misc/ri_to_c  mask(ri_to_c){}
      mask help:
      | Concatenates real and imaginary inputs into a complex output.
      | Useful for simplifying interconnects.
      | See also: Complex to Real-Imag (c_to_ri)
      mask Help: eval('xlWeb(''http://casper.berkeley.edu/wiki/Ri_to_c'')')
  sync_out : Outport
  pol0_out : Outport  Port=2
  pol1_out : Outport  Port=3
  pol2_out : Outport  Port=4
  pol3_out : Outport  Port=5
  of : Outport  Port=6
  wires:
  pol0_debus/1(msb_lsb_out1) -> pol0_out/1
  pol0_in/1 -> ri_to_c0/1(re)
  pol1_in/1 -> ri_to_c0/2(im)
  ri_to_c0/1(c) -> even_bussify/1(in1)
  pol1_debus/1(msb_lsb_out1) -> pol1_out/1
  pol2_debus/1(msb_lsb_out1) -> pol2_out/1
  pol2_in/1 -> ri_to_c1/1(re)
  pol3_in/1 -> ri_to_c1/2(im)
  ri_to_c1/1(c) -> odd_bussify/1(in1)
  pol3_debus/1(msb_lsb_out1) -> pol3_out/1
  sync/1 -> biplex_core/1(sync)
  shift/1 -> biplex_core/2(shift)
  even_bussify/1(bus_out) -> biplex_core/3(pol1)
  odd_bussify/1(bus_out) -> biplex_core/4(pol2)
  biplex_core/4(of) -> of/1
  biplex_core/1(sync_out) -> bi_real_unscr_4x/1(sync)
  biplex_core/2(out1) -> bi_real_unscr_4x/2(even)
  biplex_core/3(out2) -> bi_real_unscr_4x/3(odd)
  bi_real_unscr_4x/1(sync_out) -> sync_out/1
  bi_real_unscr_4x/2(pol1_out) -> pol0_debus/1(bus_in)
  bi_real_unscr_4x/3(pol2_out) -> pol1_debus/1(bus_in)
  bi_real_unscr_4x/4(pol3_out) -> pol2_debus/1(bus_in)
  bi_real_unscr_4x/5(pol4_out) -> pol3_debus/1(bus_in)

== system adc16_single_chan/gateway ==
  data : Inport
  Bus Creator : BusCreator  Inputs=16
  Bus Selector : BusSelector  OutputSignals=a1,a2,a3,a4
  Bus Selector1 : BusSelector  OutputSignals=b1,b2,b3,b4
  Bus Selector2 : BusSelector  OutputSignals=c1,c2,c3,c4
  Bus Selector3 : BusSelector  OutputSignals=d1,d2,d3,d4
  Gateway Out{,1..15} (16 alike) : xbsIndex_r4/Gateway Out  inherit_from_input=off  hdl_port=on  timing_constraint=None  locs_specified=off  LOCs={}  UseAsDAC=off  DACChannel='1'  block_type=gatewayout
  to_scope : Outport
  wires:
  data/1 -> Bus Selector3/1, Bus Selector2/1, Bus Selector1/1, Bus Selector/1
  Bus Selector3/4 -> Gateway Out13/1  "<d4>"
  Bus Selector3/3 -> Gateway Out12/1  "<d3>"
  Bus Selector3/2 -> Gateway Out15/1  "<d2>"
  Bus Selector3/1 -> Gateway Out14/1  "<d1>"
  Bus Selector2/4 -> Gateway Out11/1  "<c4>"
  Bus Selector2/3 -> Gateway Out10/1  "<c3>"
  Bus Selector2/2 -> Gateway Out9/1  "<c2>"
  Bus Selector2/1 -> Gateway Out8/1  "<c1>"
  Bus Selector1/2 -> Gateway Out5/1  "<b2>"
  Bus Selector1/1 -> Gateway Out4/1  "<b1>"
  Bus Selector1/4 -> Gateway Out7/1  "<b4>"
  Bus Selector1/3 -> Gateway Out6/1  "<b3>"
  Bus Selector/4 -> Gateway Out3/1  "<a4>"
  Bus Selector/2 -> Gateway Out1/1  "<a2>"
  Bus Selector/1 -> Gateway Out/1  "<a1>"
  Bus Selector/3 -> Gateway Out2/1  "<a3>"
  Bus Creator/1 -> to_scope/1
  Gateway Out4/1 -> Bus Creator/5
  Gateway Out11/1 -> Bus Creator/12
  Gateway Out10/1 -> Bus Creator/11
  Gateway Out5/1 -> Bus Creator/6
  Gateway Out9/1 -> Bus Creator/10
  Gateway Out6/1 -> Bus Creator/7
  Gateway Out8/1 -> Bus Creator/9
  Gateway Out13/1 -> Bus Creator/16
  Gateway Out/1 -> Bus Creator/1
  Gateway Out7/1 -> Bus Creator/8
  Gateway Out1/1 -> Bus Creator/2
  Gateway Out12/1 -> Bus Creator/15
  Gateway Out15/1 -> Bus Creator/14
  Gateway Out2/1 -> Bus Creator/3
  Gateway Out3/1 -> Bus Creator/4
  Gateway Out14/1 -> Bus Creator/13

== system adc16_single_chan/gateway1 ==
  data : Inport
  Bus Creator : BusCreator  Inputs=16
  Bus Selector : BusSelector  OutputSignals=signal1,signal2,signal3,signal4,signal5,signal6,signal7,signal8,signal9,signal10,signal11,signal12,signal13,signal14,signal15,signal16
  Gateway Out{,1..15} (16 alike) : xbsIndex_r4/Gateway Out  inherit_from_input=off  hdl_port=on  timing_constraint=None  locs_specified=off  LOCs={}  UseAsDAC=off  DACChannel='1'  block_type=gatewayout
  to_scope : Outport
  wires:
  Gateway Out14/1 -> Bus Creator/13
  Gateway Out3/1 -> Bus Creator/4
  Gateway Out2/1 -> Bus Creator/3
  Gateway Out15/1 -> Bus Creator/14
  Gateway Out12/1 -> Bus Creator/15
  Gateway Out1/1 -> Bus Creator/2
  Gateway Out7/1 -> Bus Creator/8
  Gateway Out/1 -> Bus Creator/1
  Gateway Out13/1 -> Bus Creator/16
  Gateway Out8/1 -> Bus Creator/9
  Gateway Out6/1 -> Bus Creator/7
  Gateway Out9/1 -> Bus Creator/10
  Gateway Out5/1 -> Bus Creator/6
  Gateway Out10/1 -> Bus Creator/11
  Gateway Out11/1 -> Bus Creator/12
  Gateway Out4/1 -> Bus Creator/5
  Bus Creator/1 -> to_scope/1
  Bus Selector/3 -> Gateway Out2/1  "<signal3>"
  Bus Selector/1 -> Gateway Out/1  "<signal1>"
  Bus Selector/2 -> Gateway Out1/1  "<signal2>"
  Bus Selector/4 -> Gateway Out3/1  "<signal4>"
  Bus Selector/7 -> Gateway Out6/1  "<signal7>"
  Bus Selector/8 -> Gateway Out7/1  "<signal8>"
  Bus Selector/5 -> Gateway Out4/1  "<signal5>"
  Bus Selector/6 -> Gateway Out5/1  "<signal6>"
  Bus Selector/9 -> Gateway Out8/1  "<signal9>"
  Bus Selector/10 -> Gateway Out9/1  "<signal10>"
  Bus Selector/11 -> Gateway Out10/1  "<signal11>"
  Bus Selector/12 -> Gateway Out11/1  "<signal12>"
  Bus Selector/13 -> Gateway Out14/1  "<signal13>"
  Bus Selector/14 -> Gateway Out15/1  "<signal14>"
  Bus Selector/15 -> Gateway Out12/1  "<signal15>"
  Bus Selector/16 -> Gateway Out13/1  "<signal16>"
  data/1 -> Bus Selector/1

== system adc16_single_chan/gateway2 ==
  data : Inport
  Bus Creator : BusCreator  Inputs=16
  Bus Selector : BusSelector  OutputSignals=signal1,signal2,signal3,signal4,signal5,signal6,signal7,signal8,signal9,signal10,signal11,signal12,signal13,signal14,signal15,signal16
  Gateway Out{,1..15} (16 alike) : xbsIndex_r4/Gateway Out  inherit_from_input=off  hdl_port=on  timing_constraint=None  locs_specified=off  LOCs={}  UseAsDAC=off  DACChannel='1'  block_type=gatewayout
  to_scope : Outport
  wires:
  data/1 -> Bus Selector/1
  Bus Selector/16 -> Gateway Out13/1  "<signal16>"
  Bus Selector/15 -> Gateway Out12/1  "<signal15>"
  Bus Selector/14 -> Gateway Out15/1  "<signal14>"
  Bus Selector/13 -> Gateway Out14/1  "<signal13>"
  Bus Selector/12 -> Gateway Out11/1  "<signal12>"
  Bus Selector/11 -> Gateway Out10/1  "<signal11>"
  Bus Selector/10 -> Gateway Out9/1  "<signal10>"
  Bus Selector/9 -> Gateway Out8/1  "<signal9>"
  Bus Selector/6 -> Gateway Out5/1  "<signal6>"
  Bus Selector/5 -> Gateway Out4/1  "<signal5>"
  Bus Selector/8 -> Gateway Out7/1  "<signal8>"
  Bus Selector/7 -> Gateway Out6/1  "<signal7>"
  Bus Selector/4 -> Gateway Out3/1  "<signal4>"
  Bus Selector/2 -> Gateway Out1/1  "<signal2>"
  Bus Selector/1 -> Gateway Out/1  "<signal1>"
  Bus Selector/3 -> Gateway Out2/1  "<signal3>"
  Bus Creator/1 -> to_scope/1
  Gateway Out4/1 -> Bus Creator/5
  Gateway Out11/1 -> Bus Creator/12
  Gateway Out10/1 -> Bus Creator/11
  Gateway Out5/1 -> Bus Creator/6
  Gateway Out9/1 -> Bus Creator/10
  Gateway Out6/1 -> Bus Creator/7
  Gateway Out8/1 -> Bus Creator/9
  Gateway Out13/1 -> Bus Creator/16
  Gateway Out/1 -> Bus Creator/1
  Gateway Out7/1 -> Bus Creator/8
  Gateway Out1/1 -> Bus Creator/2
  Gateway Out12/1 -> Bus Creator/15
  Gateway Out15/1 -> Bus Creator/14
  Gateway Out2/1 -> Bus Creator/3
  Gateway Out3/1 -> Bus Creator/4
  Gateway Out14/1 -> Bus Creator/13

== system adc16_single_chan/hold_data ==
  signals : Inport
  en : Inport  Port=2
  Bus Creator1 : BusCreator  Inputs=16
  Bus Selector : BusSelector  OutputSignals=signal1,signal2,signal3,signal4,signal5,signal6,signal7,signal8,signal9,signal10,signal11,signal12,signal13,signal14,signal15,signal16
  power_integrator : Subsystem
  power_integrator1 : Subsystem
  power_integrator10 : Subsystem
  power_integrator11 : Subsystem
  power_integrator12 : Subsystem
  power_integrator13 : Subsystem
  power_integrator14 : Subsystem
  power_integrator15 : Subsystem
  power_integrator2 : Subsystem
  power_integrator3 : Subsystem
  power_integrator4 : Subsystem
  power_integrator5 : Subsystem
  power_integrator6 : Subsystem
  power_integrator7 : Subsystem
  power_integrator8 : Subsystem
  power_integrator9 : Subsystem
  powers : Outport
  wires:
  Bus Selector/16 -> power_integrator15/1(data)  "<signal16>"
  Bus Selector/15 -> power_integrator14/1(data)  "<signal15>"
  Bus Selector/14 -> power_integrator13/1(data)  "<signal14>"
  Bus Selector/13 -> power_integrator12/1(data)  "<signal13>"
  Bus Selector/12 -> power_integrator11/1(data)  "<signal12>"
  Bus Selector/11 -> power_integrator10/1(data)  "<signal11>"
  Bus Selector/10 -> power_integrator9/1(data)  "<signal10>"
  Bus Selector/9 -> power_integrator8/1(data)  "<signal9>"
  Bus Selector/8 -> power_integrator7/1(data)  "<signal8>"
  Bus Selector/7 -> power_integrator6/1(data)  "<signal7>"
  Bus Selector/6 -> power_integrator5/1(data)  "<signal6>"
  Bus Selector/5 -> power_integrator4/1(data)  "<signal5>"
  power_integrator4/1(pow) -> Bus Creator1/5
  power_integrator1/1(pow) -> Bus Creator1/2
  power_integrator5/1(pow) -> Bus Creator1/6
  power_integrator6/1(pow) -> Bus Creator1/7
  power_integrator2/1(pow) -> Bus Creator1/3
  power_integrator7/1(pow) -> Bus Creator1/8
  power_integrator3/1(pow) -> Bus Creator1/4
  Bus Selector/4 -> power_integrator3/1(data)  "<signal4>"
  Bus Selector/3 -> power_integrator2/1(data)  "<signal3>"
  Bus Selector/2 -> power_integrator1/1(data)  "<signal2>"
  Bus Selector/1 -> power_integrator/1(data)  "<signal1>"
  Bus Creator1/1 -> powers/1
  signals/1 -> Bus Selector/1
  power_integrator/1(pow) -> Bus Creator1/1
  power_integrator11/1(pow) -> Bus Creator1/12
  power_integrator8/1(pow) -> Bus Creator1/9
  power_integrator14/1(pow) -> Bus Creator1/15
  power_integrator12/1(pow) -> Bus Creator1/13
  power_integrator15/1(pow) -> Bus Creator1/16
  power_integrator10/1(pow) -> Bus Creator1/11
  power_integrator9/1(pow) -> Bus Creator1/10
  power_integrator13/1(pow) -> Bus Creator1/14
  en/1 -> power_integrator/2(en), power_integrator1/2(en), power_integrator2/2(en), power_integrator3/2(en), power_integrator4/2(en), power_integrator5/2(en), power_integrator6/2(en), power_integrator7/2(en), power_integrator8/2(en), power_integrator9/2(en), power_integrator10/2(en), power_integrator11/2(en), power_integrator12/2(en), power_integrator13/2(en), power_integrator14/2(en), power_integrator15/2(en)
